simulink model "Chp06Code02"  (R2019a)
settings: Solver=FixedStepAuto  StartTime=0.0  StopTime=0.5  FixedStep=0.00001  RelTol=1e-3
settings Model: Creator=zhug  LastModifiedBy=ME456

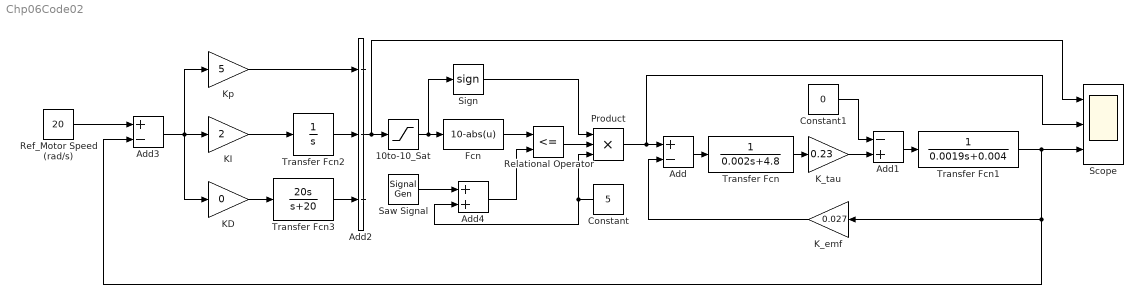
== system Chp06Code02 ==
  10to-10_Sat : Saturate  UpperLimit=10  LowerLimit=-10
  Add : Sum  Inputs=+-
  Add1 : Sum  Inputs=-+
  Add2 : Sum  Inputs=+++
  Add3 : Sum  Inputs=+-
  Add4 : Sum
  Constant : Constant  Value=5
  Constant1 : Constant  Value=0
  Fcn : Fcn  Expr=10-abs(u)
  KD : Gain  Gain=0
  KI : Gain  Gain=2
  K_emf : Gain  Gain=0.027
  K_tau : Gain  Gain=0.23
  Kp : Gain  Gain=5
  Product : Product  Inputs=3
  Ref_Motor Speed (rad/s) : Constant  Value=20
  Relational Operator : RelationalOperator  Operator=<=  OutDataTypeStr=boolean  RndMeth=Simplest
  Saw Signal : SignalGenerator  WaveForm=sawtooth  Amplitude=5  Frequency=500
  Scope : Scope  NumInputPorts=3
  Sign : Signum
  Transfer Fcn : TransferFcn  Denominator=[0.002 4.8]
  Transfer Fcn1 : TransferFcn  Denominator=[0.0019 0.004]
  Transfer Fcn2 : TransferFcn  Denominator=[1 0]
  Transfer Fcn3 : TransferFcn  Numerator=[20 0]  Denominator=[1 20]
  wires:
  Constant1/1 -> Add1/1
  KI/1 -> Transfer Fcn2/1
  Kp/1 -> Add2/1
  Add2/1 -> Scope/1, 10to-10_Sat/1
  Relational Operator/1 -> Product/2
  Add3/1 -> KD/1, Kp/1, KI/1
  Add4/1 -> Relational Operator/2
  Fcn/1 -> Relational Operator/1
  Product/1 -> Scope/2, Add/1
  Transfer Fcn2/1 -> Add2/2
  Transfer Fcn1/1 -> K_emf/1, Add3/2, Scope/3
  Add/1 -> Transfer Fcn/1
  K_tau/1 -> Add1/2
  Constant/1 -> Add4/2, Product/3
  Transfer Fcn/1 -> K_tau/1
  Saw Signal/1 -> Add4/1
  KD/1 -> Transfer Fcn3/1
  K_emf/1 -> Add/2
  10to-10_Sat/1 -> Sign/1, Fcn/1
  Add1/1 -> Transfer Fcn1/1
  Transfer Fcn3/1 -> Add2/3
  Sign/1 -> Product/1
  Ref_Motor Speed (rad/s)/1 -> Add3/1
